simulink model "PatientModelOL_DL"  (R2019a)
settings: Solver=VariableStepAuto  StartTime=0.0  StopTime=24*60  RelTol=1e-3
model workspace (MAT data in the model file):
  Cden = Simulink.Parameter
  Cden.Value = [0 0 0 0 0 0 0 0 0 1]
  Cden.DataType = 'auto'
  Cden.Dimensions = [1 10]
  Cnum = Simulink.Parameter
  Cnum.Value = [0 0 0 0 0 0 0 0 0 1]
  Cnum.DataType = 'auto'
  Cnum.Dimensions = [1 10]
  params = Simulink.Parameter
  params.Value = [1822.77593749 19.589264499 0.00675909631391 157.235805526 0.668100276788 0.00818364432629 0 15.2249530578 99.9370462412 162.365574015 157.1942967 0 0 0 0 0 0 0 0 0]
  params.DataType = 'auto'
  params.Dimensions = [1 20]
settings Model: Creator=vjoukov  LastModifiedBy=rajp0001
settings DataIOCC: ReturnWorkspaceOutputs=off
settings DebuggingCC: PregeneratedLibrarySubsystemCodeDiagnostic=none  ArithmeticOperatorsInVariantConditions=warning
settings SFSimCC: SimUseLocalCustomCode=off
settings RTWCC: RTWUseLocalCustomCode=off

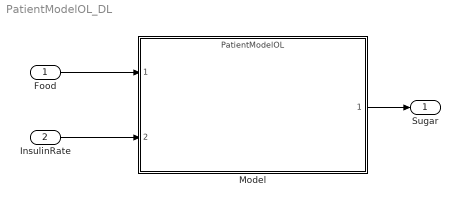
== system PatientModelOL_DL ==
  Food : Inport
  InsulinRate : Inport  Port=2
  Model : ModelReference  ModelNameDialog=PatientModelOL.slxp  ParameterArgumentNames=params  ParameterArgumentValues=params  UsingDefaultArgumentValue=0  ModelReferenceVersion=1.387  CopyOfModelProtected=on
  Sugar : Outport
  wires:
  Food/1 -> Model/1
  InsulinRate/1 -> Model/2
  Model/1 -> Sugar/1
